simulink model "memristor_subsystem"  (R2015a)
settings: Solver=ode23t  StartTime=0.0  StopTime=1.0  RelTol=1e-3
libraries: fl_lib x6, nesl_utility x5, simulink x1
settings Model: Creator=tomas  LastModifiedBy=tomas

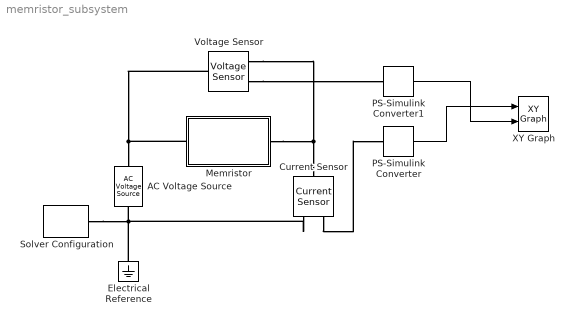
== system memristor_subsystem ==
  AC Voltage Source : fl_lib/Electrical/Electrical Sources/AC Voltage Source  amp=1 V  shift=0 deg  frequency=10 Hz  omega=0 rad/s
  Current Sensor : fl_lib/Electrical/Electrical Sensors/Current Sensor
  Electrical Reference : fl_lib/Electrical/Electrical Elements/Electrical Reference
  Memristor : Subsystem  Tag=Memristor
  PS-Simulink Converter : nesl_utility/PS-Simulink Converter  PhysicalDomain=network_engine_domain  SubClassName=ps_output  LeftPortType=input  RightPortType=output  PseudoPeriodic=off  Frequencies=[]  Unit=1  AffineConversion=off
  PS-Simulink Converter1 : nesl_utility/PS-Simulink Converter  PhysicalDomain=network_engine_domain  SubClassName=ps_output  LeftPortType=input  RightPortType=output  PseudoPeriodic=off  Frequencies=[]  Unit=1  AffineConversion=off
  Solver Configuration : nesl_utility/Solver Configuration  PhysicalDomain=network_engine_domain  SubClassName=solver  LeftPortType=input  RightPortType=generic  Accelerate=off  Tones=[]  Harmonics=[]  SimulateNoise=off  Profile=off  UseLocalSampling=off  EnableSwitchedLinearOptims=on  FrequencyDomain=off  UseCCode=off  RelTol=0.001  AbsTol=1e-06  MinStep=1e-09  ToWorkspace=off  RevertToSquareIcSolve=off  NumHomotopyIterations=100  DoDC=off  ResidualTolerance=1e-09  UseLocalSolver=off  LocalSolverChoice=NE_BACKWARD_EULER_ADVANCER  LocalSolverSampleTime=0.001  DoFixedCost=off  MaxNonlinIter=3  MaxModeIter=2  LinearAlgebra=Sparse  DelaysMemoryBudget=1024  AutomaticFiltering=on  FilteringTimeConstant=0.001
  Voltage Sensor : fl_lib/Electrical/Electrical Sensors/Voltage Sensor
  XY Graph : simulink/Sinks/XY Graph  xmin=-0.0002  xmax=0.0002  ymin=-2  ymax=2  st=-1
  wires:
  PS-Simulink Converter1/1 -> XY Graph/2
  PS-Simulink Converter/1 -> XY Graph/1
  connections:
  Memristor/LConn1 -- Voltage Sensor/LConn1 -- AC Voltage Source/LConn1
  AC Voltage Source/RConn1 -- Current Sensor/RConn2 -- Solver Configuration/RConn1 -- Electrical Reference/LConn1
  Memristor/RConn1 -- Voltage Sensor/RConn2 -- Current Sensor/LConn1
  Current Sensor/RConn1 -- PS-Simulink Converter/LConn1
  Voltage Sensor/RConn1 -- PS-Simulink Converter1/LConn1

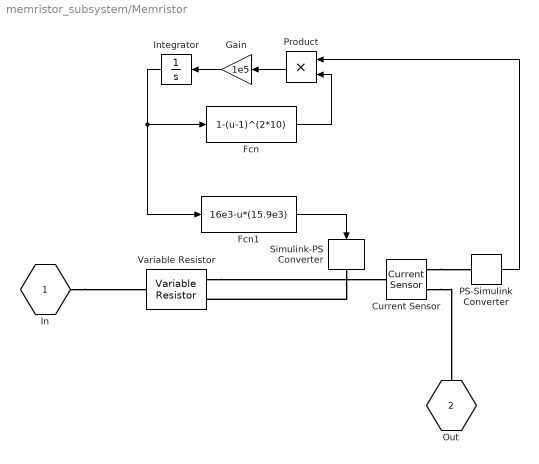
== system memristor_subsystem/Memristor ==
  Current Sensor : fl_lib/Electrical/Electrical Sensors/Current Sensor
  Fcn : Fcn  Expr=1-(u-1)^(2*10)
  Fcn1 : Fcn  Expr=16e3-u*(15.9e3)
  Gain : Gain  Gain=1e5
  Integrator : Integrator  InitialCondition=0.3145
  PS-Simulink Converter : nesl_utility/PS-Simulink Converter  PhysicalDomain=network_engine_domain  SubClassName=ps_output  LeftPortType=input  RightPortType=output  PseudoPeriodic=off  Frequencies=[]  Unit=1  AffineConversion=off
  Product : Product
  Simulink-PS Converter : nesl_utility/Simulink-PS Converter  PhysicalDomain=network_engine_domain  SubClassName=ps_input  LeftPortType=input  RightPortType=output  PseudoPeriodic=off  Frequencies=[]  NoiseDistribution=none  NoiseParameters=[]  Unit=1  AffineConversion=off  InputFiltering=off  SimscapeFilterOrder=1  InputFilterTimeConstant=0.001  UdotUserProvided=1
  Variable Resistor : fl_lib/Electrical/Electrical Elements/Variable Resistor  Rmin=0 Ohm  i_specify=off  i_priority=High  i=0 A  v_specify=off  v_priority=High  v=0 V
  In : PMIOPort  Port=1  Side=Left
  Out : PMIOPort  Port=2  Side=Right
  wires:
  Gain/1 -> Integrator/1
  Product/1 -> Gain/1
  Integrator/1 -> Fcn1/1, Fcn/1
  Fcn/1 -> Product/2
  Fcn1/1 -> Simulink-PS Converter/1
  PS-Simulink Converter/1 -> Product/1
  connections:
  In/RConn1 -- Variable Resistor/RConn1
  Variable Resistor/LConn2 -- Current Sensor/LConn1
  Current Sensor/RConn1 -- PS-Simulink Converter/LConn1
  Simulink-PS Converter/RConn1 -- Variable Resistor/LConn1
  Current Sensor/RConn2 -- Out/RConn1
